simulink model "omniwheel_standard"  (R2023b)
settings: Solver=VariableStepAuto  StartTime=0.0  StopTime=10.0  RelTol=1e-3
undefined symbols (not defined in the file): sampleTime
libraries: mobileRoboticsLib x4
settings Model: Creator=mihai  LastModifiedBy=mihai

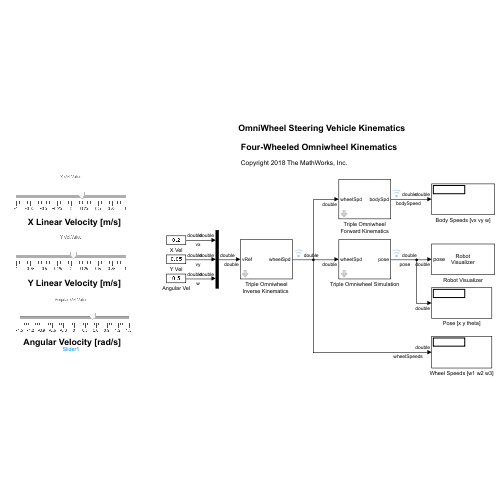
[thumbnail: Simulink's stored preview of the top-level diagram]
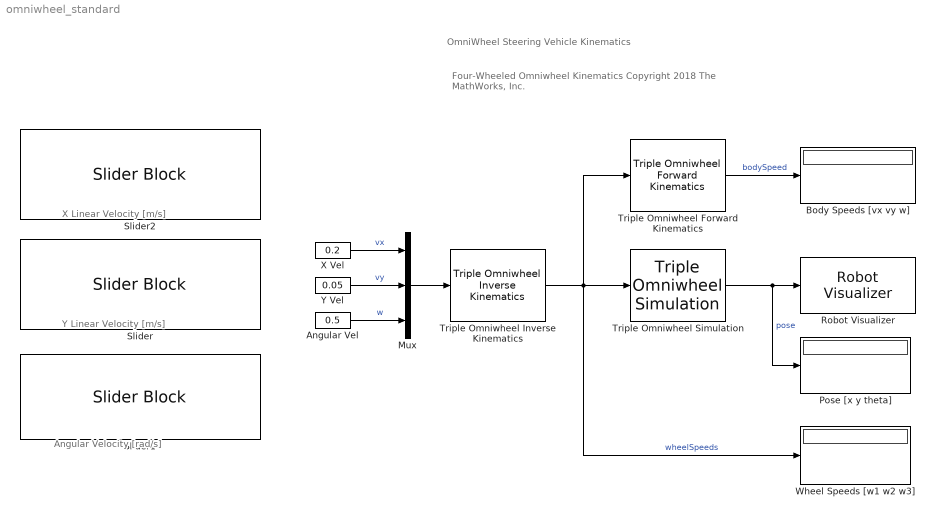
== system omniwheel_standard ==
  note: OmniWheel Steering Vehicle Kinematics
  note: X Linear Velocity [m/s]
  note: Four-Wheeled Omniwheel Kinematics
      |
      | Copyright 2018 The MathWorks, Inc.
  note: Angular Velocity [rad/s]
  note: Y Linear Velocity [m/s]
  Angular Vel : Constant  Value=0.5
  Body Speeds [vx vy w] : Display
  Mux : Mux  Inputs=3
  Pose [x y theta] : Display
  Robot Visualizer : mobileRoboticsLib/Environments/Robot Visualizer  Priority=99  robotRadius=0  showTrajectory=on  hasWaypoints=off  hasLidar=off  sensorOffset=[ 0 0 ]  scanAngles=scanAngles  hasObjDetector=off  objDetectorOffset=[ 0, 0 ]  objDetectorAngle=0  objDetectorFOV=pi/4  objDetectorMaxRange=5  objectColors=[ 1, 0, 0; 0, 1, 0; 0, 0, 1 ]  objectMarkers=s
  Slider : SliderBlock  ScaleMin=-1  ScaleMax=1  TickInterval=0.25
  Slider1 : SliderBlock  ScaleMin=-1.5  ScaleMax=1.5
  Slider2 : SliderBlock  ScaleMin=-1  ScaleMax=1  TickInterval=0.25
  Triple Omniwheel Forward Kinematics : mobileRoboticsLib/Kinematic Models/Triple Omniwheel/Triple Omniwheel Forward Kinematics  wheelRadius=wheelRadius  robotRadius=robotRadius  wheelAngles=wheelAngles
      settings: SourceProductName=Mobile Robotics Simulation Toolbox
  "Triple Omniwheel Inverse Kinematics " : mobileRoboticsLib/Kinematic Models/Triple Omniwheel/Triple Omniwheel Inverse Kinematics   wheelRadius=wheelRadius  robotRadius=robotRadius  wheelAngles=wheelAngles
      settings: SourceProductName=Mobile Robotics Simulation Toolbox
  Triple Omniwheel Simulation : mobileRoboticsLib/Kinematic Models/Triple Omniwheel/Triple Omniwheel Simulation  wheelRadius=wheelRadius  robotRadius=robotRadius  wheelAngles=wheelAngles  initX=0  initY=0  initAngle=0  Ts=sampleTime
      settings: SourceProductName=Mobile Robotics Simulation Toolbox
  Wheel Speeds [w1 w2 w3] : Display
  X Vel : Constant  Value=0.2
  Y Vel : Constant  Value=0.05
  wires:
  X Vel/1 -> Mux/1  "vx"
  "Triple Omniwheel Inverse Kinematics "/1 -> Triple Omniwheel Forward Kinematics/1, Triple Omniwheel Simulation/1, Wheel Speeds [w1 w2 w3]/1  "wheelSpeeds"
  Triple Omniwheel Forward Kinematics/1 -> Body Speeds [vx vy w]/1  "bodySpeed"
  Mux/1 -> "Triple Omniwheel Inverse Kinematics "/1
  Triple Omniwheel Simulation/1 -> Pose [x y theta]/1, Robot Visualizer/1  "pose"
  Angular Vel/1 -> Mux/3  "w"
  Y Vel/1 -> Mux/2  "vy"
